simulink model "example_algorithm_mappings"  (R2016a)
settings: Solver=VariableStepAuto  StartTime=0.0  StopTime=10.0  RelTol=1e-3
libraries: simulink x3
settings Model: Creator=mgreiff  LastModifiedBy=mgreiff

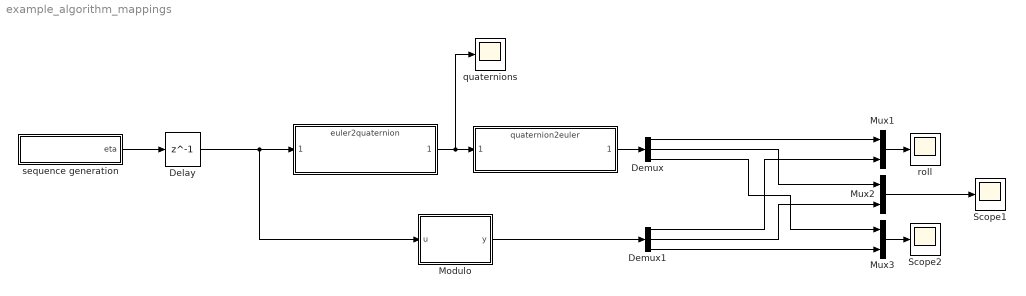
== system example_algorithm_mappings ==
  " " : ModelReference  ModelNameDialog=quaternion2euler.mdl  SimulationMode=Normal  ModelReferenceVersion=1.92
  "   " : ModelReference  ModelNameDialog=euler2quaternion.mdl  SimulationMode=Normal  ModelReferenceVersion=1.5
  Delay : Delay  DelayLength=1  InitialCondition=0  SampleTime=0.01
  Demux : Demux  Outputs=3
  Demux1 : Demux  Outputs=3
  Modulo : MATLAB Function  TreatAsAtomicUnit=on
  Mux1 : Mux  Inputs=2
  Mux2 : Mux  Inputs=2
  Mux3 : Mux  Inputs=2
  Scope1 : Scope
  Scope2 : Scope
  quaternions : Scope
  roll : Scope
  sequence generation : Subsystem
  wires:
  "   "/1 -> quaternions/1, " "/1
  Demux/1 -> Mux1/1
  Demux/2 -> Mux2/1
  Demux/3 -> Mux3/1
  Mux1/1 -> roll/1
  Mux2/1 -> Scope1/1
  Mux3/1 -> Scope2/1
  sequence generation/1(eta) -> Delay/1
  Demux1/1 -> Mux1/2
  Demux1/3 -> Mux3/2
  Demux1/2 -> Mux2/2
  Modulo/1(y) -> Demux1/1
  " "/1 -> Demux/1
  Delay/1 -> "   "/1, Modulo/1(u)

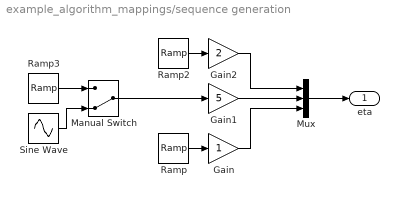
== system example_algorithm_mappings/sequence generation ==
  Gain : Gain
  Gain1 : Gain  Gain=5
  Gain2 : Gain  Gain=2
  Manual Switch : ManualSwitch  CurrentSetting=0
  Mux : Mux  Inputs=3
  Ramp : simulink/Sources/Ramp  slope=1  start=0  X0=0
  Ramp2 : simulink/Sources/Ramp  slope=1  start=0  X0=0
  Ramp3 : simulink/Sources/Ramp  slope=1  start=0  X0=0
  Sine Wave : Sin  SampleTime=0
  eta : Outport
  wires:
  Sine Wave/1 -> Manual Switch/2
  Ramp2/1 -> Gain2/1
  Gain2/1 -> Mux/1
  Gain/1 -> Mux/3
  Manual Switch/1 -> Gain1/1
  Ramp3/1 -> Manual Switch/1
  Gain1/1 -> Mux/2
  Ramp/1 -> Gain/1
  Mux/1 -> eta/1

== matlab function example_algorithm_mappings/Modulo ==
  data: u input; y output
function y = fcn(u)
%#codegen
y = mod(u, 2*pi);
